simulink model "ModeloExperimentalyTeorico"  (R2023b)
settings: Solver=VariableStepAuto  StartTime=0.0  StopTime=10.0  RelTol=1e-3
settings Model: Creator=USUARIO  LastModifiedBy=USUARIO

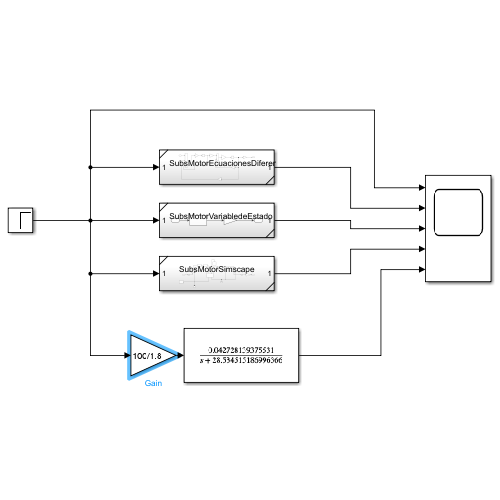
[thumbnail: Simulink's stored preview of the top-level diagram]
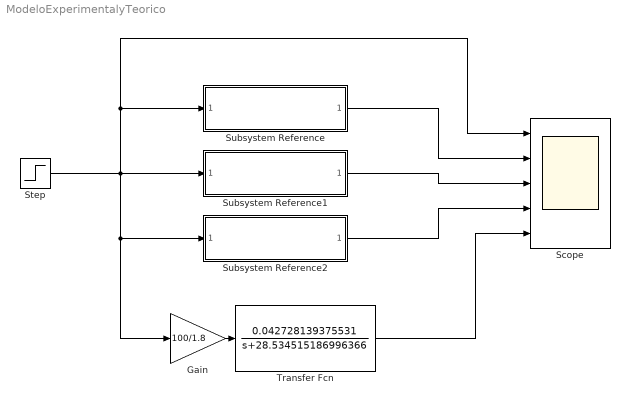
== system ModeloExperimentalyTeorico ==
  Gain : Gain  Gain=100/1.8
  Scope : Scope  NumInputPorts=5
  Step : Step  After=5  SampleTime=0
  Subsystem Reference : Subsystem  ReferencedSubsystem=SubsMotorEcuacionesDiferenciales
  Subsystem Reference1 : Subsystem  ReferencedSubsystem=SubsMotorVariabledeEstado
  Subsystem Reference2 : Subsystem  ReferencedSubsystem=SubsMotorSimscape
  Transfer Fcn : TransferFcn  Numerator=[0.042728139375531]  Denominator=[1 28.534515186996366]
  wires:
  Gain/1 -> Transfer Fcn/1
  Step/1 -> Gain/1, Subsystem Reference2/1, Subsystem Reference/1, Scope/1, Subsystem Reference1/1
  Subsystem Reference/1 -> Scope/2
  Subsystem Reference1/1 -> Scope/3
  Subsystem Reference2/1 -> Scope/4
  Transfer Fcn/1 -> Scope/5
